simulink model "model_moj"  (R2024a)
settings: Solver=VariableStepAuto  StartTime=0.0  StopTime=400  RelTol=1e-3
undefined symbols (not defined in the file): National_Instruments, PCIe, t_step_t, t_step_v, up_nominalna, ut_1, ut_2, ut_nominalna, uv_1, uv_2
libraries: sldrtlib x4
settings Model: Creator=lab  LastModifiedBy=slowepoke
settings DebuggingCC: UnconnectedInputMsg=warning  UnconnectedOutputMsg=warning  UnconnectedLineMsg=warning
settings ModelReferenceCC: EnableRefExpFcnMdlSchedulingChecks=on
settings RTWCC: GPUComputeCapability=3.5  DLArmComputeVersion=19.05

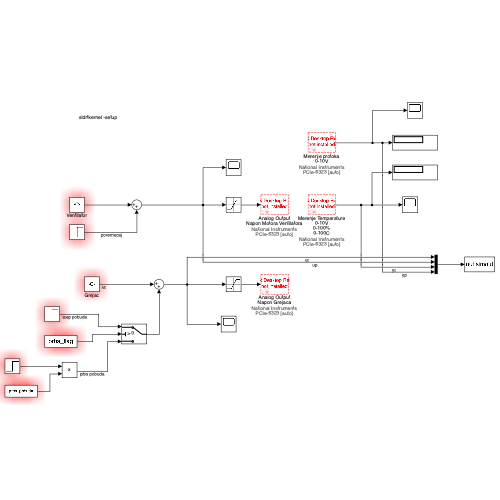
[thumbnail: Simulink's stored preview of the top-level diagram]
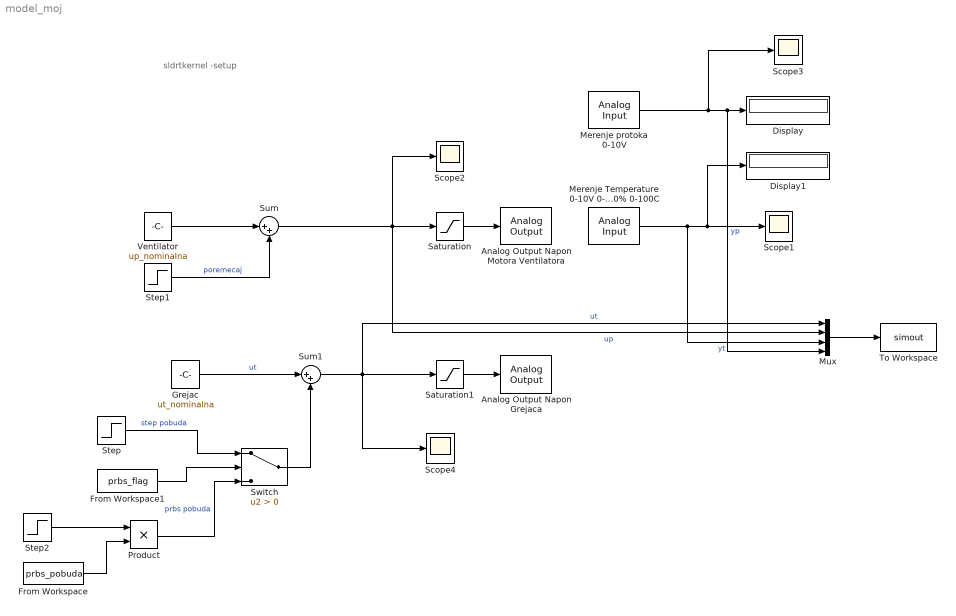
== system model_moj ==
  note: sldrtkernel -setup
  Analog Output Napon Grejaca : sldrtlib/Analog Output  SampleTime=0.01  MaxMissedTicks=10000  ShowMissedTicks=off  YieldWhenWaiting=off  DrvName=National_Instruments/PCIe-6323  DrvAddress=4294967295  DrvOptions=[0 0 0 0 0 0 0]  Channels=2  RangeMode=1  VoltRange=1  InitialValue=0  FinalValue=0
      settings: AttributesFormatString=National Instruments\nPCIe-6323 [auto]
  Analog Output Napon Motora Ventilatora : sldrtlib/Analog Output  SampleTime=0.01  MaxMissedTicks=10000  ShowMissedTicks=off  YieldWhenWaiting=off  DrvName=National_Instruments/PCIe-6323  DrvAddress=4294967295  DrvOptions=[0 0 0 0 0 0 0]  Channels=1  RangeMode=1  VoltRange=1  InitialValue=[]  FinalValue=[]
      settings: AttributesFormatString=National Instruments\nPCIe-6323 [auto]
  Display : Display
  Display1 : Display
  From Workspace : FromWorkspace  VariableName=prbs_pobuda
  From Workspace1 : FromWorkspace  VariableName=prbs_flag
  Grejac : Constant  Value=ut_nominalna
  Merenje Temperature 0-10V 0-100% 0-100C : sldrtlib/Analog Input  SampleTime=0.01  MaxMissedTicks=10000  ShowMissedTicks=off  YieldWhenWaiting=off  DrvName=National_Instruments/PCIe-6323  DrvAddress=4294967295  DrvOptions=[0 0 0 0 0 0 0]  Channels=3  RangeMode=1  VoltRange=1  DataType=1
      settings: AttributesFormatString=National Instruments\nPCIe-6323 [auto]
  Merenje protoka 0-10V : sldrtlib/Analog Input  SampleTime=0.01  MaxMissedTicks=10000  ShowMissedTicks=off  YieldWhenWaiting=on  DrvName=National_Instruments/PCIe-6323  DrvAddress=4294967295  DrvOptions=[0 0 0 0 0 0 0]  Channels=6  RangeMode=1  VoltRange=1  DataType=1
      settings: AttributesFormatString=National Instruments\nPCIe-6323 [auto]
  Mux : Mux
  Product : Product
  Saturation : Saturate  UpperLimit=10  LowerLimit=0
  Saturation1 : Saturate  UpperLimit=10  LowerLimit=0
  Scope{1..4} (4 alike) : Scope
  Step : Step  Time=t_step_t  Before=ut_1  After=ut_2  SampleTime=0
  Step1 : Step  Time=t_step_v  Before=uv_1  After=uv_2  SampleTime=0
  Step2 : Step  Time=t_step_t  SampleTime=0
  Sum : Sum  Inputs=|++
  Sum1 : Sum  Inputs=|++
  Switch : Switch  Criteria=u2 > Threshold  SaturateOnIntegerOverflow=off  InputSameDT=off
  To Workspace : ToWorkspace  VariableName=simout  SampleTime=0.01
  Ventilator : Constant  Value=up_nominalna
  wires:
  Grejac/1 -> Sum1/1  "ut"
  Mux/1 -> To Workspace/1
  Saturation1/1 -> Analog Output Napon Grejaca/1
  Merenje protoka 0-10V/1 -> Display/1, Mux/4, Scope3/1  "yp"
  Saturation/1 -> Analog Output Napon Motora Ventilatora/1
  Ventilator/1 -> Sum/1
  Merenje Temperature 0-10V 0-100% 0-100C/1 -> Mux/3, Display1/1, Scope1/1  "yt"
  Step1/1 -> Sum/2  "poremecaj"
  Sum/1 -> Saturation/1, Mux/2, Scope2/1  "up"
  Sum1/1 -> Mux/1, Scope4/1, Saturation1/1  "ut"
  Step2/1 -> Product/1
  From Workspace/1 -> Product/2
  Step/1 -> Switch/1  "step pobuda"
  Product/1 -> Switch/3  "prbs pobuda"
  Switch/1 -> Sum1/2
  From Workspace1/1 -> Switch/2
